simulink library "HardwareCommunication"  (R2016b)
settings: Solver=VariableStepAuto  StartTime=0.0  StopTime=10.0  RelTol=1e-3
undefined symbols (not defined in the file or in its folder): EthercatDeviceError
libraries: inSOMANET x28, SendToSOMANET x28, VariousLibrary x14, GESHandler x8, InputDeviceHandler x8, PDBHandler x8, SOMANETHandler x8, xpcethercatlib x7, ReceiveFromInputDevice x7, ReceiveFromGES x7, ReceiveFromPDB x7, SendToInputDevice x7
(part 1 of 2)
settings Model: Creator=march  LastModifiedBy=march

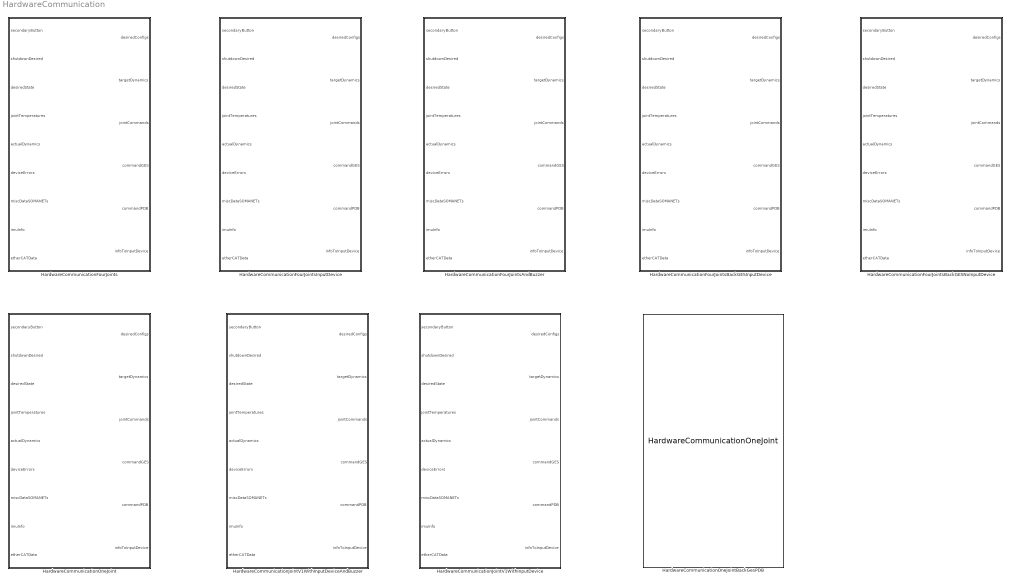
== system HardwareCommunication ==
  HardwareCommunicationFourJoints : Subsystem
  HardwareCommunicationFourJointsAndBuzzer : Subsystem
  HardwareCommunicationFourJointsBackGESInputDevice : Subsystem
  HardwareCommunicationFourJointsBackGESNoInputDevice : Subsystem
  HardwareCommunicationFourJointsInputDevice : Subsystem
  HardwareCommunicationJointV1WithInputDevice : Subsystem
  HardwareCommunicationJointV1WithInputDeviceAndBuzzer : Subsystem
  HardwareCommunicationOneJoint : Subsystem
  HardwareCommunicationOneJointBackGesPDB : HardwareCommunication/HardwareCommunicationOneJoint

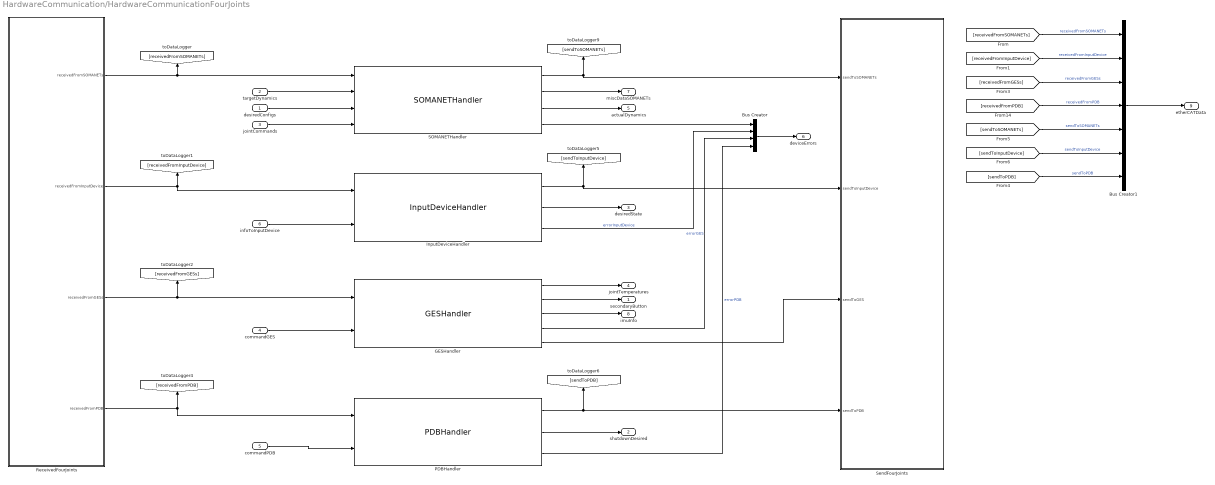
== system HardwareCommunication/HardwareCommunicationFourJoints ==
  desiredConfigs : Inport
  targetDynamics : Inport  Port=2
  jointCommands : Inport  Port=3
  commandGES : Inport  Port=4  OutDataTypeStr=Bus: commandGES
  commandPDB : Inport  Port=5
  infoToInputDevice : Inport  Port=6
  Bus Creator : BusCreator  Inputs=4  OutDataTypeStr=Bus: DeviceErrors  NonVirtualBus=on
  Bus Creator1 : BusCreator  Inputs=7  OutDataTypeStr=Bus: EtherCATData  NonVirtualBus=on
  GESHandler : GESHandler/GESHandler
  InputDeviceHandler : InputDeviceHandler/InputDeviceHandler
  PDBHandler : PDBHandler/PDBHandler
  ReceivedFourJoints : Subsystem
  SOMANETHandler : SOMANETHandler/SOMANETHandler
  SendFourJoints : Subsystem
  secondaryButton : Outport
  shutdownDesired : Outport  Port=2
  desiredState : Outport  Port=3
  jointTemperatures : Outport  Port=4
  actualDynamics : Outport  Port=5
  deviceErrors : Outport  Port=6
  miscDataSOMANETs : Outport  Port=7
  imuInfo : Outport  Port=8
  etherCATData : Outport  Port=9
  wires:
  GESHandler/5 -> SendFourJoints/3(sendToGES)
  infoToInputDevice/1 -> InputDeviceHandler/2
  ReceivedFourJoints/3(receivedFromGESs) -> GESHandler/1, [receivedFromGESs]
  ReceivedFourJoints/2(receivedFromInputDevice) -> InputDeviceHandler/1, [receivedFromInputDevice]
  ReceivedFourJoints/4(receivedFromPDB) -> PDBHandler/1, [receivedFromPDB]
  InputDeviceHandler/1 -> SendFourJoints/2(sendToInputDevice), [sendToInputDevice]
  InputDeviceHandler/3 -> Bus Creator/2  "errorInputDevice"
  Bus Creator/1 -> deviceErrors/1
  PDBHandler/1 -> SendFourJoints/4(sendToPDB), [sendToPDB]
  [receivedFromInputDevice] -> Bus Creator1/2  "receivedFromInputDevice"
  [receivedFromSOMANETs] -> Bus Creator1/1  "receivedFromSOMANETs"
  SOMANETHandler/2 -> miscDataSOMANETs/1
  [sendToPDB] -> Bus Creator1/7  "sendToPDB"
  ReceivedFourJoints/1(receivedFromSOMANETs) -> [receivedFromSOMANETs], SOMANETHandler/1
  GESHandler/2 -> secondaryButton/1
  SOMANETHandler/1 -> SendFourJoints/1(sendToSOMANETs), [sendToSOMANETs]
  InputDeviceHandler/2 -> desiredState/1
  jointCommands/1 -> SOMANETHandler/4
  SOMANETHandler/3 -> actualDynamics/1
  [sendToSOMANETs] -> Bus Creator1/5  "sendToSOMANETs"
  [sendToInputDevice] -> Bus Creator1/6  "sendToInputDevice"
  [receivedFromGESs] -> Bus Creator1/3  "receivedFromGESs"
  SOMANETHandler/4 -> Bus Creator/1
  desiredConfigs/1 -> SOMANETHandler/3
  [receivedFromPDB] -> Bus Creator1/4  "receivedFromPDB"
  Bus Creator1/1 -> etherCATData/1
  GESHandler/1 -> jointTemperatures/1
  PDBHandler/3 -> Bus Creator/4  "errorPDB"
  commandGES/1 -> GESHandler/2
  GESHandler/4 -> Bus Creator/3  "errorGES"
  commandPDB/1 -> PDBHandler/2
  PDBHandler/2 -> shutdownDesired/1
  targetDynamics/1 -> SOMANETHandler/2
  GESHandler/3 -> imuInfo/1

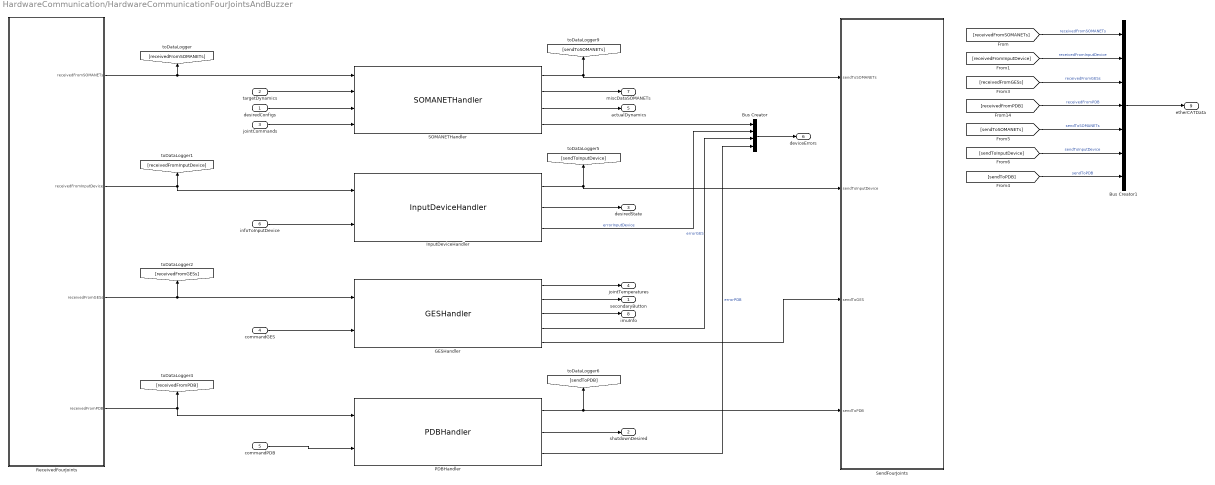
== system HardwareCommunication/HardwareCommunicationFourJointsAndBuzzer ==
  desiredConfigs : Inport
  targetDynamics : Inport  Port=2
  jointCommands : Inport  Port=3
  commandGES : Inport  Port=4
  commandPDB : Inport  Port=5
  infoToInputDevice : Inport  Port=6
  Bus Creator : BusCreator  Inputs=4  OutDataTypeStr=Bus: DeviceErrors  NonVirtualBus=on
  Bus Creator1 : BusCreator  Inputs=7  OutDataTypeStr=Bus: EtherCATData  NonVirtualBus=on
  GESHandler : GESHandler/GESHandler
  InputDeviceHandler : InputDeviceHandler/InputDeviceHandler
  PDBHandler : PDBHandler/PDBHandler
  ReceivedFourJoints : Subsystem
  SOMANETHandler : SOMANETHandler/SOMANETHandler
  SendFourJoints : Subsystem
  secondaryButton : Outport
  shutdownDesired : Outport  Port=2
  desiredState : Outport  Port=3
  jointTemperatures : Outport  Port=4
  actualDynamics : Outport  Port=5
  deviceErrors : Outport  Port=6
  miscDataSOMANETs : Outport  Port=7
  imuInfo : Outport  Port=8
  etherCATData : Outport  Port=9
  wires:
  GESHandler/5 -> SendFourJoints/3(sendToGES)
  infoToInputDevice/1 -> InputDeviceHandler/2
  ReceivedFourJoints/3(receivedFromGESs) -> GESHandler/1, [receivedFromGESs]
  ReceivedFourJoints/2(receivedFromInputDevice) -> InputDeviceHandler/1, [receivedFromInputDevice]
  ReceivedFourJoints/4(receivedFromPDB) -> PDBHandler/1, [receivedFromPDB]
  InputDeviceHandler/1 -> SendFourJoints/2(sendToInputDevice), [sendToInputDevice]
  InputDeviceHandler/3 -> Bus Creator/2  "errorInputDevice"
  Bus Creator/1 -> deviceErrors/1
  PDBHandler/1 -> SendFourJoints/4(sendToPDB), [sendToPDB]
  [receivedFromInputDevice] -> Bus Creator1/2  "receivedFromInputDevice"
  [receivedFromSOMANETs] -> Bus Creator1/1  "receivedFromSOMANETs"
  SOMANETHandler/2 -> miscDataSOMANETs/1
  [sendToPDB] -> Bus Creator1/7  "sendToPDB"
  ReceivedFourJoints/1(receivedFromSOMANETs) -> [receivedFromSOMANETs], SOMANETHandler/1
  GESHandler/2 -> secondaryButton/1
  SOMANETHandler/1 -> SendFourJoints/1(sendToSOMANETs), [sendToSOMANETs]
  InputDeviceHandler/2 -> desiredState/1
  jointCommands/1 -> SOMANETHandler/4
  SOMANETHandler/3 -> actualDynamics/1
  [sendToSOMANETs] -> Bus Creator1/5  "sendToSOMANETs"
  [sendToInputDevice] -> Bus Creator1/6  "sendToInputDevice"
  [receivedFromGESs] -> Bus Creator1/3  "receivedFromGESs"
  SOMANETHandler/4 -> Bus Creator/1
  desiredConfigs/1 -> SOMANETHandler/3
  [receivedFromPDB] -> Bus Creator1/4  "receivedFromPDB"
  Bus Creator1/1 -> etherCATData/1
  GESHandler/1 -> jointTemperatures/1
  PDBHandler/3 -> Bus Creator/4  "errorPDB"
  commandGES/1 -> GESHandler/2
  GESHandler/4 -> Bus Creator/3  "errorGES"
  commandPDB/1 -> PDBHandler/2
  PDBHandler/2 -> shutdownDesired/1
  targetDynamics/1 -> SOMANETHandler/2
  GESHandler/3 -> imuInfo/1

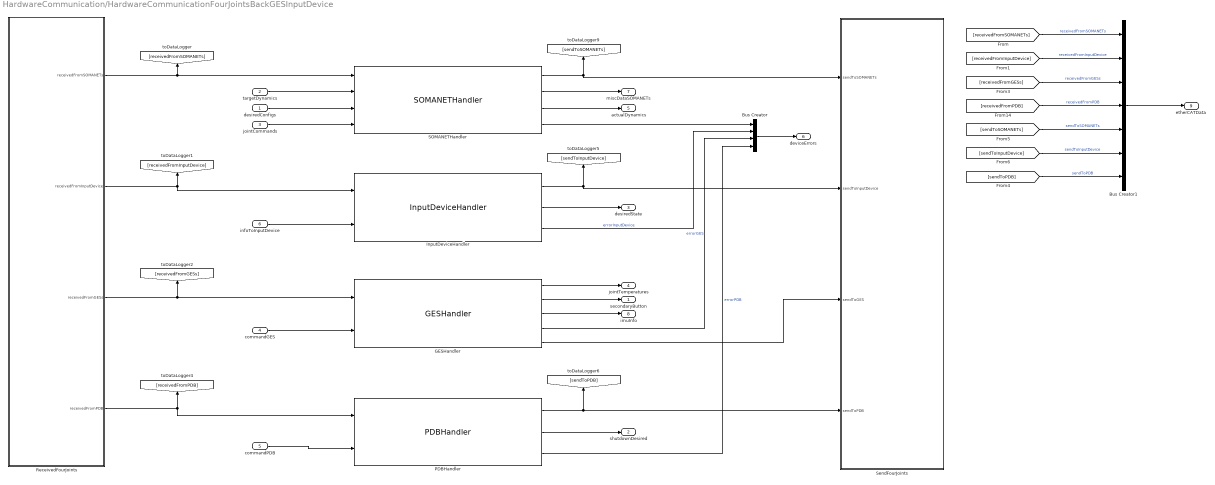
== system HardwareCommunication/HardwareCommunicationFourJointsBackGESInputDevice ==
  desiredConfigs : Inport
  targetDynamics : Inport  Port=2
  jointCommands : Inport  Port=3
  commandGES : Inport  Port=4
  commandPDB : Inport  Port=5
  infoToInputDevice : Inport  Port=6
  Bus Creator : BusCreator  Inputs=4  OutDataTypeStr=Bus: DeviceErrors  NonVirtualBus=on
  Bus Creator1 : BusCreator  Inputs=7  OutDataTypeStr=Bus: EtherCATData  NonVirtualBus=on
  GESHandler : GESHandler/GESHandler
  InputDeviceHandler : InputDeviceHandler/InputDeviceHandler
  PDBHandler : PDBHandler/PDBHandler
  ReceivedFourJoints : Subsystem
  SOMANETHandler : SOMANETHandler/SOMANETHandler
  SendFourJoints : Subsystem
  secondaryButton : Outport
  shutdownDesired : Outport  Port=2
  desiredState : Outport  Port=3
  jointTemperatures : Outport  Port=4
  actualDynamics : Outport  Port=5
  deviceErrors : Outport  Port=6
  miscDataSOMANETs : Outport  Port=7
  imuInfo : Outport  Port=8
  etherCATData : Outport  Port=9
  wires:
  GESHandler/3 -> imuInfo/1
  targetDynamics/1 -> SOMANETHandler/2
  PDBHandler/2 -> shutdownDesired/1
  commandPDB/1 -> PDBHandler/2
  GESHandler/4 -> Bus Creator/3  "errorGES"
  commandGES/1 -> GESHandler/2
  PDBHandler/3 -> Bus Creator/4  "errorPDB"
  GESHandler/1 -> jointTemperatures/1
  Bus Creator1/1 -> etherCATData/1
  [receivedFromPDB] -> Bus Creator1/4  "receivedFromPDB"
  desiredConfigs/1 -> SOMANETHandler/3
  SOMANETHandler/4 -> Bus Creator/1
  [receivedFromGESs] -> Bus Creator1/3  "receivedFromGESs"
  [sendToInputDevice] -> Bus Creator1/6  "sendToInputDevice"
  [sendToSOMANETs] -> Bus Creator1/5  "sendToSOMANETs"
  SOMANETHandler/3 -> actualDynamics/1
  jointCommands/1 -> SOMANETHandler/4
  InputDeviceHandler/2 -> desiredState/1
  SOMANETHandler/1 -> [sendToSOMANETs], SendFourJoints/1(sendToSOMANETs)
  GESHandler/2 -> secondaryButton/1
  ReceivedFourJoints/1(receivedFromSOMANETs) -> SOMANETHandler/1, [receivedFromSOMANETs]
  [sendToPDB] -> Bus Creator1/7  "sendToPDB"
  SOMANETHandler/2 -> miscDataSOMANETs/1
  [receivedFromSOMANETs] -> Bus Creator1/1  "receivedFromSOMANETs"
  [receivedFromInputDevice] -> Bus Creator1/2  "receivedFromInputDevice"
  PDBHandler/1 -> [sendToPDB], SendFourJoints/4(sendToPDB)
  Bus Creator/1 -> deviceErrors/1
  InputDeviceHandler/3 -> Bus Creator/2  "errorInputDevice"
  InputDeviceHandler/1 -> [sendToInputDevice], SendFourJoints/2(sendToInputDevice)
  ReceivedFourJoints/4(receivedFromPDB) -> [receivedFromPDB], PDBHandler/1
  ReceivedFourJoints/2(receivedFromInputDevice) -> [receivedFromInputDevice], InputDeviceHandler/1
  ReceivedFourJoints/3(receivedFromGESs) -> [receivedFromGESs], GESHandler/1
  infoToInputDevice/1 -> InputDeviceHandler/2
  GESHandler/5 -> SendFourJoints/3(sendToGES)

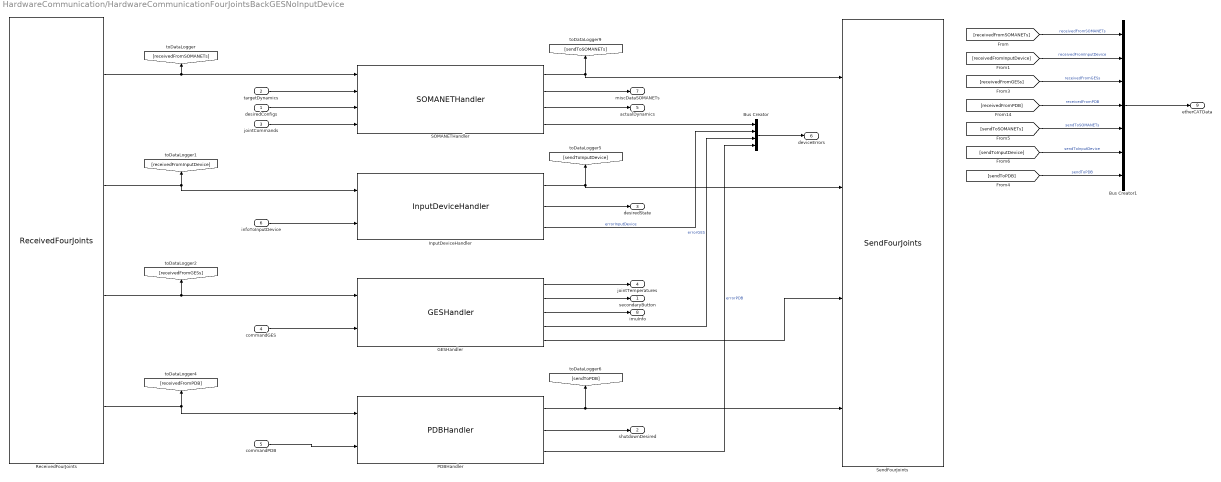
== system HardwareCommunication/HardwareCommunicationFourJointsBackGESNoInputDevice ==
  desiredConfigs : Inport
  targetDynamics : Inport  Port=2
  jointCommands : Inport  Port=3
  commandGES : Inport  Port=4
  commandPDB : Inport  Port=5
  infoToInputDevice : Inport  Port=6
  Bus Creator : BusCreator  Inputs=4  OutDataTypeStr=Bus: DeviceErrors  NonVirtualBus=on
  Bus Creator1 : BusCreator  Inputs=7  OutDataTypeStr=Bus: EtherCATData  NonVirtualBus=on
  GESHandler : GESHandler/GESHandler
  InputDeviceHandler : InputDeviceHandler/InputDeviceHandler
  PDBHandler : PDBHandler/PDBHandler
  ReceivedFourJoints : HardwareCommunication/HardwareCommunicationFourJointsBackGESInputDevice/ReceivedFourJoints
  SOMANETHandler : SOMANETHandler/SOMANETHandler
  SendFourJoints : HardwareCommunication/HardwareCommunicationFourJointsBackGESInputDevice/SendFourJoints
  secondaryButton : Outport
  shutdownDesired : Outport  Port=2
  desiredState : Outport  Port=3
  jointTemperatures : Outport  Port=4
  actualDynamics : Outport  Port=5
  deviceErrors : Outport  Port=6
  miscDataSOMANETs : Outport  Port=7
  imuInfo : Outport  Port=8
  etherCATData : Outport  Port=9
  wires:
  Bus Creator1/1 -> etherCATData/1
  desiredConfigs/1 -> SOMANETHandler/3
  SOMANETHandler/4 -> Bus Creator/1
  [receivedFromGESs] -> Bus Creator1/3  "receivedFromGESs"
  [receivedFromPDB] -> Bus Creator1/4  "receivedFromPDB"
  [sendToInputDevice] -> Bus Creator1/6  "sendToInputDevice"
  [sendToSOMANETs] -> Bus Creator1/5  "sendToSOMANETs"
  PDBHandler/3 -> Bus Creator/4  "errorPDB"
  SOMANETHandler/3 -> actualDynamics/1
  PDBHandler/2 -> shutdownDesired/1
  commandPDB/1 -> PDBHandler/2
  targetDynamics/1 -> SOMANETHandler/2
  GESHandler/4 -> Bus Creator/3  "errorGES"
  GESHandler/3 -> imuInfo/1
  commandGES/1 -> GESHandler/2
  GESHandler/1 -> jointTemperatures/1
  [receivedFromInputDevice] -> Bus Creator1/2  "receivedFromInputDevice"
  InputDeviceHandler/2 -> desiredState/1
  SOMANETHandler/1 -> [sendToSOMANETs], SendFourJoints/1
  InputDeviceHandler/1 -> [sendToInputDevice], SendFourJoints/2
  GESHandler/2 -> secondaryButton/1
  ReceivedFourJoints/2 -> [receivedFromInputDevice], InputDeviceHandler/1
  SOMANETHandler/2 -> miscDataSOMANETs/1
  PDBHandler/1 -> [sendToPDB], SendFourJoints/4
  [sendToPDB] -> Bus Creator1/7  "sendToPDB"
  Bus Creator/1 -> deviceErrors/1
  InputDeviceHandler/3 -> Bus Creator/2  "errorInputDevice"
  ReceivedFourJoints/4 -> [receivedFromPDB], PDBHandler/1
  GESHandler/5 -> SendFourJoints/3
  infoToInputDevice/1 -> InputDeviceHandler/2
  jointCommands/1 -> SOMANETHandler/4
  [receivedFromSOMANETs] -> Bus Creator1/1  "receivedFromSOMANETs"
  ReceivedFourJoints/1 -> SOMANETHandler/1, [receivedFromSOMANETs]
  ReceivedFourJoints/3 -> [receivedFromGESs], GESHandler/1

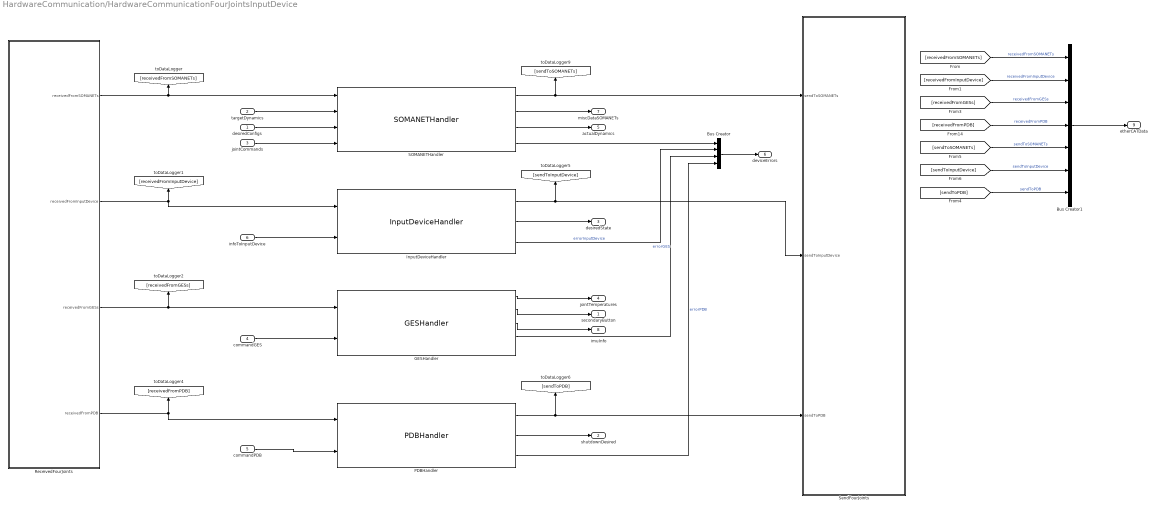
== system HardwareCommunication/HardwareCommunicationFourJointsInputDevice ==
  desiredConfigs : Inport
  targetDynamics : Inport  Port=2
  jointCommands : Inport  Port=3
  commandGES : Inport  Port=4
  commandPDB : Inport  Port=5
  infoToInputDevice : Inport  Port=6
  Bus Creator : BusCreator  Inputs=4  OutDataTypeStr=Bus: DeviceErrors  NonVirtualBus=on
  Bus Creator1 : BusCreator  Inputs=7  OutDataTypeStr=Bus: EtherCATData  NonVirtualBus=on
  GESHandler : GESHandler/GESHandler
  InputDeviceHandler : InputDeviceHandler/InputDeviceHandler
  PDBHandler : PDBHandler/PDBHandler
  ReceivedFourJoints : Subsystem
  SOMANETHandler : SOMANETHandler/SOMANETHandler
  SendFourJoints : Subsystem
  secondaryButton : Outport
  shutdownDesired : Outport  Port=2
  desiredState : Outport  Port=3
  jointTemperatures : Outport  Port=4
  actualDynamics : Outport  Port=5
  deviceErrors : Outport  Port=6
  miscDataSOMANETs : Outport  Port=7
  imuInfo : Outport  Port=8
  etherCATData : Outport  Port=9
  wires:
  GESHandler/3 -> imuInfo/1
  targetDynamics/1 -> SOMANETHandler/2
  PDBHandler/2 -> shutdownDesired/1
  commandPDB/1 -> PDBHandler/2
  GESHandler/4 -> Bus Creator/3  "errorGES"
  commandGES/1 -> GESHandler/2
  PDBHandler/3 -> Bus Creator/4  "errorPDB"
  GESHandler/1 -> jointTemperatures/1
  Bus Creator1/1 -> etherCATData/1
  [receivedFromPDB] -> Bus Creator1/4  "receivedFromPDB"
  desiredConfigs/1 -> SOMANETHandler/3
  SOMANETHandler/4 -> Bus Creator/1
  [receivedFromGESs] -> Bus Creator1/3  "receivedFromGESs"
  [sendToInputDevice] -> Bus Creator1/6  "sendToInputDevice"
  [sendToSOMANETs] -> Bus Creator1/5  "sendToSOMANETs"
  SOMANETHandler/3 -> actualDynamics/1
  jointCommands/1 -> SOMANETHandler/4
  InputDeviceHandler/2 -> desiredState/1
  SOMANETHandler/1 -> [sendToSOMANETs], SendFourJoints/1(sendToSOMANETs)
  GESHandler/2 -> secondaryButton/1
  ReceivedFourJoints/1(receivedFromSOMANETs) -> SOMANETHandler/1, [receivedFromSOMANETs]
  [sendToPDB] -> Bus Creator1/7  "sendToPDB"
  SOMANETHandler/2 -> miscDataSOMANETs/1
  [receivedFromSOMANETs] -> Bus Creator1/1  "receivedFromSOMANETs"
  [receivedFromInputDevice] -> Bus Creator1/2  "receivedFromInputDevice"
  PDBHandler/1 -> [sendToPDB], SendFourJoints/3(sendToPDB)
  Bus Creator/1 -> deviceErrors/1
  InputDeviceHandler/3 -> Bus Creator/2  "errorInputDevice"
  InputDeviceHandler/1 -> [sendToInputDevice], SendFourJoints/2(sendToInputDevice)
  ReceivedFourJoints/4(receivedFromPDB) -> [receivedFromPDB], PDBHandler/1
  ReceivedFourJoints/2(receivedFromInputDevice) -> [receivedFromInputDevice], InputDeviceHandler/1
  ReceivedFourJoints/3(receivedFromGESs) -> [receivedFromGESs], GESHandler/1
  infoToInputDevice/1 -> InputDeviceHandler/2

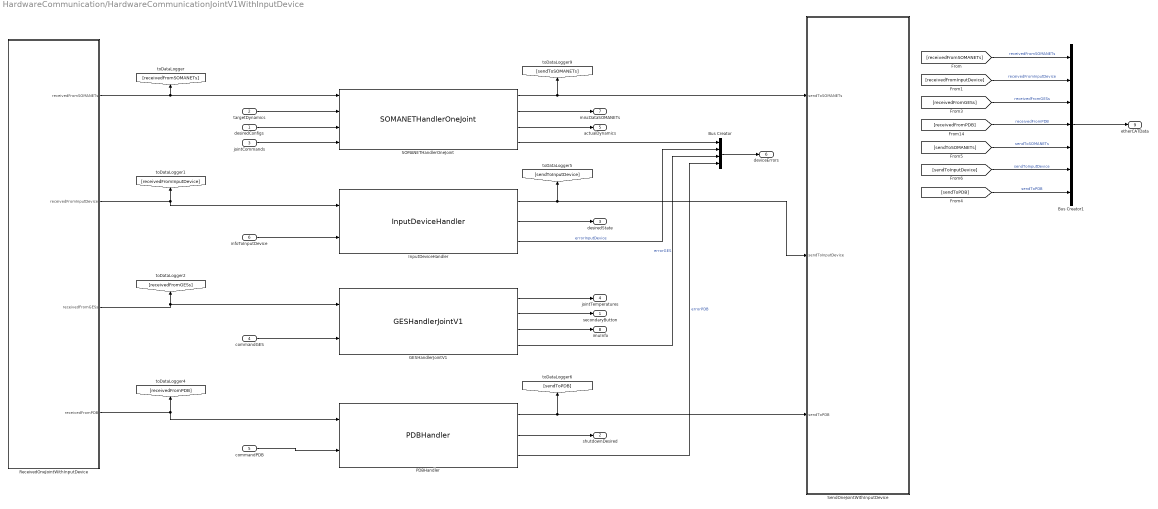
== system HardwareCommunication/HardwareCommunicationJointV1WithInputDevice ==
  desiredConfigs : Inport
  targetDynamics : Inport  Port=2
  jointCommands : Inport  Port=3
  commandGES : Inport  Port=4
  commandPDB : Inport  Port=5
  infoToInputDevice : Inport  Port=6
  Bus Creator : BusCreator  Inputs=4  OutDataTypeStr=Bus: DeviceErrors  NonVirtualBus=on
  Bus Creator1 : BusCreator  Inputs=7  OutDataTypeStr=Bus: EtherCATData  NonVirtualBus=on
  GESHandlerJointV1 : GESHandler/GESHandlerJointV1
  InputDeviceHandler : InputDeviceHandler/InputDeviceHandler
  PDBHandler : PDBHandler/PDBHandler
  ReceivedOneJointWithInputDevice : Subsystem
  SOMANETHandlerOneJoint : SOMANETHandler/SOMANETHandlerOneJoint
  SendOneJointWithInputDevice : Subsystem
  secondaryButton : Outport
  shutdownDesired : Outport  Port=2
  desiredState : Outport  Port=3
  jointTemperatures : Outport  Port=4
  actualDynamics : Outport  Port=5
  deviceErrors : Outport  Port=6
  miscDataSOMANETs : Outport  Port=7
  imuInfo : Outport  Port=8
  etherCATData : Outport  Port=9
  wires:
  infoToInputDevice/1 -> InputDeviceHandler/2
  ReceivedOneJointWithInputDevice/3(receivedFromGESs) -> [receivedFromGESs], GESHandlerJointV1/1
  ReceivedOneJointWithInputDevice/2(receivedFromInputDevice) -> InputDeviceHandler/1, [receivedFromInputDevice]
  ReceivedOneJointWithInputDevice/4(receivedFromPDB) -> PDBHandler/1, [receivedFromPDB]
  InputDeviceHandler/1 -> [sendToInputDevice], SendOneJointWithInputDevice/2(sendToInputDevice)
  InputDeviceHandler/3 -> Bus Creator/2  "errorInputDevice"
  Bus Creator/1 -> deviceErrors/1
  PDBHandler/1 -> [sendToPDB], SendOneJointWithInputDevice/3(sendToPDB)
  [receivedFromInputDevice] -> Bus Creator1/2  "receivedFromInputDevice"
  [receivedFromSOMANETs] -> Bus Creator1/1  "receivedFromSOMANETs"
  SOMANETHandlerOneJoint/2 -> miscDataSOMANETs/1
  [sendToPDB] -> Bus Creator1/7  "sendToPDB"
  ReceivedOneJointWithInputDevice/1(receivedFromSOMANETs) -> [receivedFromSOMANETs], SOMANETHandlerOneJoint/1
  GESHandlerJointV1/2 -> secondaryButton/1
  SOMANETHandlerOneJoint/1 -> [sendToSOMANETs], SendOneJointWithInputDevice/1(sendToSOMANETs)
  InputDeviceHandler/2 -> desiredState/1
  jointCommands/1 -> SOMANETHandlerOneJoint/4
  SOMANETHandlerOneJoint/3 -> actualDynamics/1
  [sendToSOMANETs] -> Bus Creator1/5  "sendToSOMANETs"
  [sendToInputDevice] -> Bus Creator1/6  "sendToInputDevice"
  [receivedFromGESs] -> Bus Creator1/3  "receivedFromGESs"
  SOMANETHandlerOneJoint/4 -> Bus Creator/1
  desiredConfigs/1 -> SOMANETHandlerOneJoint/3
  [receivedFromPDB] -> Bus Creator1/4  "receivedFromPDB"
  Bus Creator1/1 -> etherCATData/1
  GESHandlerJointV1/1 -> jointTemperatures/1
  PDBHandler/3 -> Bus Creator/4  "errorPDB"
  commandGES/1 -> GESHandlerJointV1/2
  GESHandlerJointV1/4 -> Bus Creator/3  "errorGES"
  commandPDB/1 -> PDBHandler/2
  PDBHandler/2 -> shutdownDesired/1
  targetDynamics/1 -> SOMANETHandlerOneJoint/2
  GESHandlerJointV1/3 -> imuInfo/1

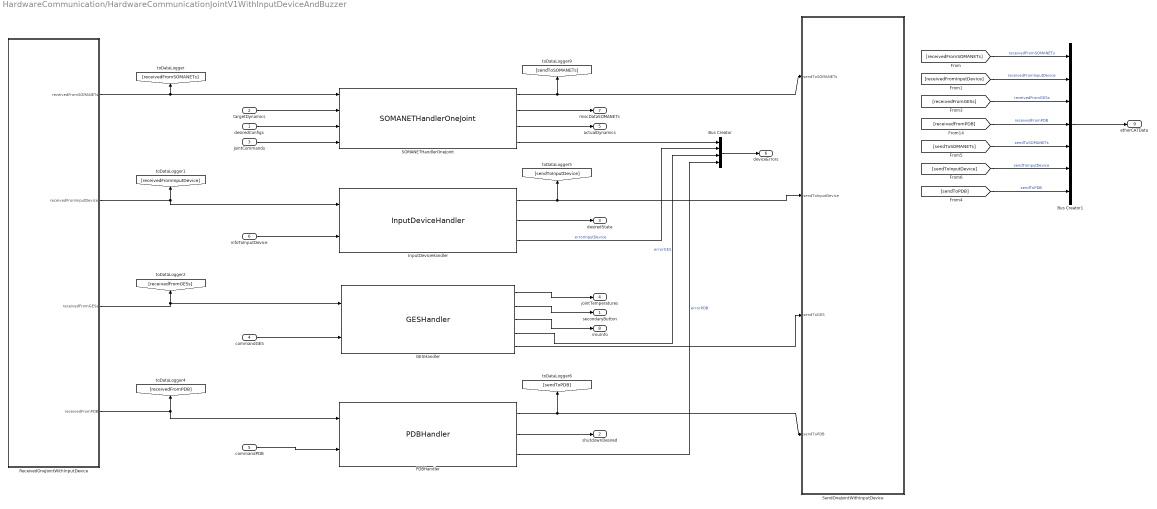
== system HardwareCommunication/HardwareCommunicationJointV1WithInputDeviceAndBuzzer ==
  desiredConfigs : Inport
  targetDynamics : Inport  Port=2
  jointCommands : Inport  Port=3
  commandGES : Inport  Port=4
  commandPDB : Inport  Port=5
  infoToInputDevice : Inport  Port=6
  Bus Creator : BusCreator  Inputs=4  OutDataTypeStr=Bus: DeviceErrors  NonVirtualBus=on
  Bus Creator1 : BusCreator  Inputs=7  OutDataTypeStr=Bus: EtherCATData  NonVirtualBus=on
  GESHandler : GESHandler/GESHandler
  InputDeviceHandler : InputDeviceHandler/InputDeviceHandler
  PDBHandler : PDBHandler/PDBHandler
  ReceivedOneJointWithInputDevice : Subsystem
  SOMANETHandlerOneJoint : SOMANETHandler/SOMANETHandlerOneJoint
  SendOneJointWithInputDevice : Subsystem
  secondaryButton : Outport
  shutdownDesired : Outport  Port=2
  desiredState : Outport  Port=3
  jointTemperatures : Outport  Port=4
  actualDynamics : Outport  Port=5
  deviceErrors : Outport  Port=6
  miscDataSOMANETs : Outport  Port=7
  imuInfo : Outport  Port=8
  etherCATData : Outport  Port=9
  wires:
  infoToInputDevice/1 -> InputDeviceHandler/2
  ReceivedOneJointWithInputDevice/3(receivedFromGESs) -> GESHandler/1, [receivedFromGESs]
  ReceivedOneJointWithInputDevice/2(receivedFromInputDevice) -> InputDeviceHandler/1, [receivedFromInputDevice]
  ReceivedOneJointWithInputDevice/4(receivedFromPDB) -> PDBHandler/1, [receivedFromPDB]
  InputDeviceHandler/1 -> [sendToInputDevice], SendOneJointWithInputDevice/2(sendToInputDevice)
  InputDeviceHandler/3 -> Bus Creator/2  "errorInputDevice"
  Bus Creator/1 -> deviceErrors/1
  PDBHandler/1 -> [sendToPDB], SendOneJointWithInputDevice/4(sendToPDB)
  [receivedFromInputDevice] -> Bus Creator1/2  "receivedFromInputDevice"
  [receivedFromSOMANETs] -> Bus Creator1/1  "receivedFromSOMANETs"
  SOMANETHandlerOneJoint/2 -> miscDataSOMANETs/1
  [sendToPDB] -> Bus Creator1/7  "sendToPDB"
  ReceivedOneJointWithInputDevice/1(receivedFromSOMANETs) -> [receivedFromSOMANETs], SOMANETHandlerOneJoint/1
  GESHandler/2 -> secondaryButton/1
  SOMANETHandlerOneJoint/1 -> [sendToSOMANETs], SendOneJointWithInputDevice/1(sendToSOMANETs)
  InputDeviceHandler/2 -> desiredState/1
  jointCommands/1 -> SOMANETHandlerOneJoint/4
  SOMANETHandlerOneJoint/3 -> actualDynamics/1
  [sendToSOMANETs] -> Bus Creator1/5  "sendToSOMANETs"
  [sendToInputDevice] -> Bus Creator1/6  "sendToInputDevice"
  [receivedFromGESs] -> Bus Creator1/3  "receivedFromGESs"
  SOMANETHandlerOneJoint/4 -> Bus Creator/1
  desiredConfigs/1 -> SOMANETHandlerOneJoint/3
  [receivedFromPDB] -> Bus Creator1/4  "receivedFromPDB"
  Bus Creator1/1 -> etherCATData/1
  GESHandler/1 -> jointTemperatures/1
  PDBHandler/3 -> Bus Creator/4  "errorPDB"
  commandGES/1 -> GESHandler/2
  GESHandler/4 -> Bus Creator/3  "errorGES"
  commandPDB/1 -> PDBHandler/2
  PDBHandler/2 -> shutdownDesired/1
  targetDynamics/1 -> SOMANETHandlerOneJoint/2
  GESHandler/3 -> imuInfo/1
  GESHandler/5 -> SendOneJointWithInputDevice/3(sendToGES)

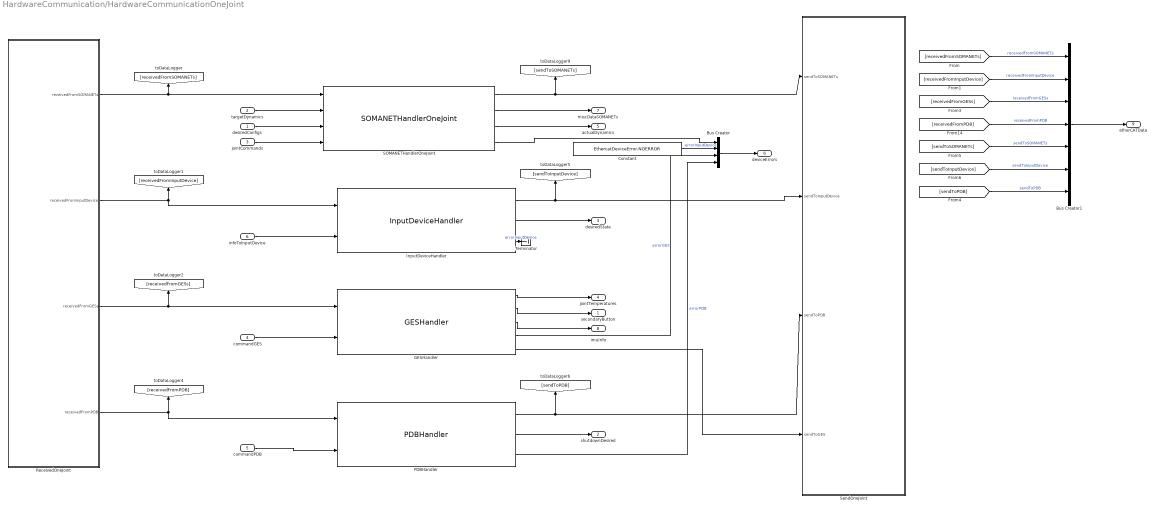
== system HardwareCommunication/HardwareCommunicationOneJoint ==
  desiredConfigs : Inport
  targetDynamics : Inport  Port=2
  jointCommands : Inport  Port=3
  commandGES : Inport  Port=4
  commandPDB : Inport  Port=5
  infoToInputDevice : Inport  Port=6
  Bus Creator : BusCreator  Inputs=4  OutDataTypeStr=Bus: DeviceErrors  NonVirtualBus=on
  Bus Creator1 : BusCreator  Inputs=7  OutDataTypeStr=Bus: EtherCATData  NonVirtualBus=on
  Constant : Constant  Value=EthercatDeviceError.NOERROR
  GESHandler : GESHandler/GESHandler
  InputDeviceHandler : InputDeviceHandler/InputDeviceHandler
  PDBHandler : PDBHandler/PDBHandler
  ReceivedOneJoint : Subsystem
  SOMANETHandlerOneJoint : SOMANETHandler/SOMANETHandlerOneJoint
  SendOneJoint : Subsystem
  Terminator : Terminator
  secondaryButton : Outport
  shutdownDesired : Outport  Port=2
  desiredState : Outport  Port=3
  jointTemperatures : Outport  Port=4
  actualDynamics : Outport  Port=5
  deviceErrors : Outport  Port=6
  miscDataSOMANETs : Outport  Port=7
  imuInfo : Outport  Port=8
  etherCATData : Outport  Port=9
  wires:
  InputDeviceHandler/3 -> Terminator/1  "errorInputDevice"
  Constant/1 -> Bus Creator/2  "errorInputDevice"
  GESHandler/5 -> SendOneJoint/4(sendToGES)
  infoToInputDevice/1 -> InputDeviceHandler/2
  ReceivedOneJoint/3(receivedFromGESs) -> GESHandler/1, [receivedFromGESs]
  ReceivedOneJoint/2(receivedFromInputDevice) -> InputDeviceHandler/1, [receivedFromInputDevice]
  ReceivedOneJoint/4(receivedFromPDB) -> PDBHandler/1, [receivedFromPDB]
  InputDeviceHandler/1 -> SendOneJoint/2(sendToInputDevice), [sendToInputDevice]
  Bus Creator/1 -> deviceErrors/1
  PDBHandler/1 -> SendOneJoint/3(sendToPDB), [sendToPDB]
  [receivedFromInputDevice] -> Bus Creator1/2  "receivedFromInputDevice"
  [receivedFromSOMANETs] -> Bus Creator1/1  "receivedFromSOMANETs"
  SOMANETHandlerOneJoint/2 -> miscDataSOMANETs/1
  [sendToPDB] -> Bus Creator1/7  "sendToPDB"
  ReceivedOneJoint/1(receivedFromSOMANETs) -> [receivedFromSOMANETs], SOMANETHandlerOneJoint/1
  GESHandler/2 -> secondaryButton/1
  SOMANETHandlerOneJoint/1 -> SendOneJoint/1(sendToSOMANETs), [sendToSOMANETs]
  InputDeviceHandler/2 -> desiredState/1
  jointCommands/1 -> SOMANETHandlerOneJoint/4
  SOMANETHandlerOneJoint/3 -> actualDynamics/1
  [sendToSOMANETs] -> Bus Creator1/5  "sendToSOMANETs"
  [sendToInputDevice] -> Bus Creator1/6  "sendToInputDevice"
  [receivedFromGESs] -> Bus Creator1/3  "receivedFromGESs"
  SOMANETHandlerOneJoint/4 -> Bus Creator/1
  desiredConfigs/1 -> SOMANETHandlerOneJoint/3
  [receivedFromPDB] -> Bus Creator1/4  "receivedFromPDB"
  Bus Creator1/1 -> etherCATData/1
  GESHandler/1 -> jointTemperatures/1
  PDBHandler/3 -> Bus Creator/4  "errorPDB"
  commandGES/1 -> GESHandler/2
  GESHandler/4 -> Bus Creator/3  "errorGES"
  commandPDB/1 -> PDBHandler/2
  PDBHandler/2 -> shutdownDesired/1
  targetDynamics/1 -> SOMANETHandlerOneJoint/2
  GESHandler/3 -> imuInfo/1

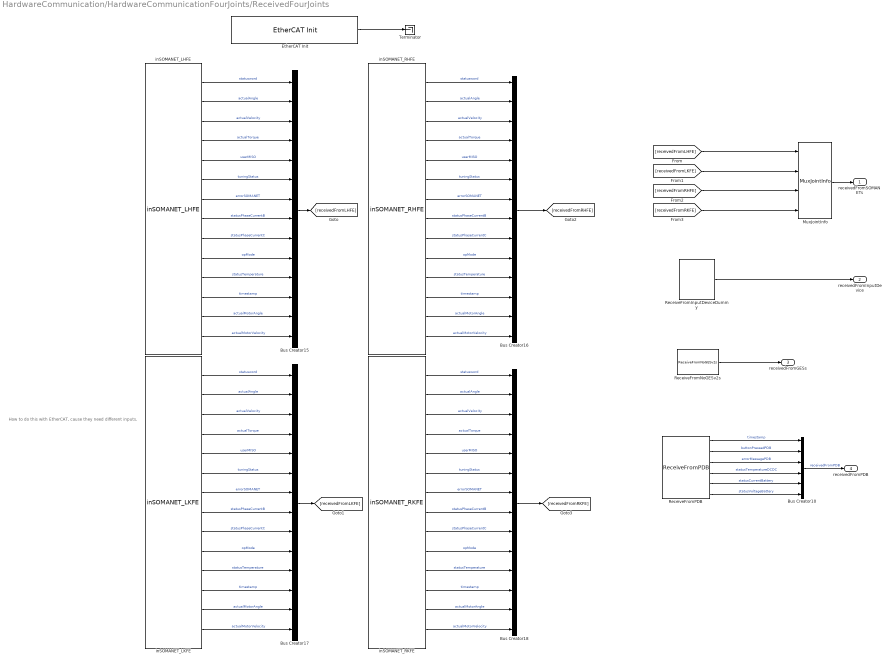
== system HardwareCommunication/HardwareCommunicationFourJoints/ReceivedFourJoints ==
  note: How to do this with EtherCAT, cause they need different inputs.
  Bus Creator10 : BusCreator  Inputs=6  OutDataTypeStr=Bus: EtherCATReceivedFromPDB  NonVirtualBus=on
  Bus Creator{15..18} (4 alike) : BusCreator  Inputs=14  OutDataTypeStr=Bus: EtherCATReceivedFromSOMANET  NonVirtualBus=on
  "EtherCAT Init " : xpcethercatlib/EtherCAT Init   Priority=0  config_file=..\EcatXML\FourJointsOnly_eni.xml  device_id=0  pci_bus=2  pci_slot=0  dctuning=0  enaDebug=on  enaDC=on  errLink=on  masterDbg=on  stateChgDbg=on  baseClock=off  masterCfg=off  logFile='c:\dbglog.txt'  sample_time=0.002000  DCMode=0
  MuxJointInfo : VariousLibrary/MuxJointInfo
  ReceiveFromInputDeviceDummy : ReceiveFromInputDevice/ReceiveFromInputDeviceDummy
  ReceiveFromNoGESv2s : ReceiveFromGES/ReceiveFromNoGESv2s
  ReceiveFromPDB : ReceiveFromPDB/ReceiveFromPDB
  Terminator : Terminator
  inSOMANET_LHFE : inSOMANET/inSOMANET_LHFE
  inSOMANET_LKFE : inSOMANET/inSOMANET_LKFE
  inSOMANET_RHFE : inSOMANET/inSOMANET_RHFE
  inSOMANET_RKFE : inSOMANET/inSOMANET_RKFE
  receivedFromSOMANETs : Outport  OutDataTypeStr=Bus: EtherCATReceivedFromSOMANET  PortDimensions=[ 1 4 ]  BusOutputAsStruct=on
  receivedFromInputDevice : Outport  Port=2  OutDataTypeStr=Bus: EtherCATReceivedFromInputDevice  BusOutputAsStruct=on
  receivedFromGESs : Outport  Port=3  OutDataTypeStr=Bus: EtherCATReceivedFromGES  PortDimensions=[1 4]  BusOutputAsStruct=on
  receivedFromPDB : Outport  Port=4  OutDataTypeStr=Bus: EtherCATReceivedFromPDB  BusOutputAsStruct=on
  wires:
  ReceiveFromPDB/1 -> Bus Creator10/1  "timestamp"
  [receivedFromLKFE] -> MuxJointInfo/2
  [receivedFromRKFE] -> MuxJointInfo/4
  [receivedFromRHFE] -> MuxJointInfo/3
  [receivedFromLHFE] -> MuxJointInfo/1
  Bus Creator18/1 -> [receivedFromRKFE]
  inSOMANET_RKFE/11 -> Bus Creator18/11  "statusTemperature"
  inSOMANET_LKFE/11 -> Bus Creator17/11  "statusTemperature"
  inSOMANET_RKFE/12 -> Bus Creator18/12  "timestamp"
  inSOMANET_RKFE/6 -> Bus Creator18/6  "tuningStatus"
  inSOMANET_RKFE/1 -> Bus Creator18/1  "statusword"
  inSOMANET_LKFE/5 -> Bus Creator17/5  "userMISO"
  inSOMANET_RKFE/7 -> Bus Creator18/7  "errorSOMANET"
  inSOMANET_RKFE/8 -> Bus Creator18/8  "statusPhaseCurrentB"
  inSOMANET_RKFE/3 -> Bus Creator18/3  "actualVelocity"
  inSOMANET_RKFE/5 -> Bus Creator18/5  "userMISO"
  inSOMANET_LKFE/8 -> Bus Creator17/8  "statusPhaseCurrentB"
  inSOMANET_LKFE/12 -> Bus Creator17/12  "timestamp"
  Bus Creator17/1 -> [receivedFromLKFE]
  inSOMANET_RKFE/10 -> Bus Creator18/10  "opMode"
  inSOMANET_LKFE/6 -> Bus Creator17/6  "tuningStatus"
  inSOMANET_LKFE/10 -> Bus Creator17/10  "opMode"
  inSOMANET_RKFE/2 -> Bus Creator18/2  "actualAngle"
  inSOMANET_RKFE/9 -> Bus Creator18/9  "statusPhaseCurrentC"
  inSOMANET_RKFE/4 -> Bus Creator18/4  "actualTorque"
  inSOMANET_LKFE/9 -> Bus Creator17/9  "statusPhaseCurrentC"
  inSOMANET_LHFE/9 -> Bus Creator15/9  "statusPhaseCurrentC"
  inSOMANET_LKFE/7 -> Bus Creator17/7  "errorSOMANET"
  inSOMANET_LKFE/4 -> Bus Creator17/4  "actualTorque"
  MuxJointInfo/1 -> receivedFromSOMANETs/1
  inSOMANET_LKFE/3 -> Bus Creator17/3  "actualVelocity"
  inSOMANET_RHFE/8 -> Bus Creator16/8  "statusPhaseCurrentB"
  inSOMANET_RHFE/5 -> Bus Creator16/5  "userMISO"
  inSOMANET_LHFE/8 -> Bus Creator15/8  "statusPhaseCurrentB"
  inSOMANET_LHFE/4 -> Bus Creator15/4  "actualTorque"
  inSOMANET_LHFE/12 -> Bus Creator15/12  "timestamp"
  inSOMANET_LKFE/2 -> Bus Creator17/2  "actualAngle"
  inSOMANET_RHFE/12 -> Bus Creator16/12  "timestamp"
  inSOMANET_LHFE/3 -> Bus Creator15/3  "actualVelocity"
  inSOMANET_LKFE/1 -> Bus Creator17/1  "statusword"
  Bus Creator16/1 -> [receivedFromRHFE]
  Bus Creator15/1 -> [receivedFromLHFE]
  inSOMANET_RHFE/11 -> Bus Creator16/11  "statusTemperature"
  inSOMANET_LHFE/7 -> Bus Creator15/7  "errorSOMANET"
  inSOMANET_RHFE/10 -> Bus Creator16/10  "opMode"
  inSOMANET_RHFE/9 -> Bus Creator16/9  "statusPhaseCurrentC"
  inSOMANET_RHFE/7 -> Bus Creator16/7  "errorSOMANET"
  inSOMANET_RHFE/1 -> Bus Creator16/1  "statusword"
  inSOMANET_LHFE/2 -> Bus Creator15/2  "actualAngle"
  inSOMANET_RHFE/6 -> Bus Creator16/6  "tuningStatus"
  inSOMANET_RHFE/4 -> Bus Creator16/4  "actualTorque"
  inSOMANET_RHFE/3 -> Bus Creator16/3  "actualVelocity"
  inSOMANET_RHFE/2 -> Bus Creator16/2  "actualAngle"
  inSOMANET_LHFE/11 -> Bus Creator15/11  "statusTemperature"
  inSOMANET_LHFE/1 -> Bus Creator15/1  "statusword"
  inSOMANET_LHFE/10 -> Bus Creator15/10  "opMode"
  inSOMANET_LHFE/6 -> Bus Creator15/6  "tuningStatus"
  Bus Creator10/1 -> receivedFromPDB/1  "receivedFromPDB"
  inSOMANET_LHFE/5 -> Bus Creator15/5  "userMISO"
  "EtherCAT Init "/1 -> Terminator/1
  inSOMANET_LHFE/13 -> Bus Creator15/13  "actualMotorAngle"
  inSOMANET_LHFE/14 -> Bus Creator15/14  "actualMotorVelocity"
  inSOMANET_LKFE/13 -> Bus Creator17/13  "actualMotorAngle"
  inSOMANET_LKFE/14 -> Bus Creator17/14  "actualMotorVelocity"
  inSOMANET_RKFE/13 -> Bus Creator18/13  "actualMotorAngle"
  inSOMANET_RKFE/14 -> Bus Creator18/14  "actualMotorVelocity"
  inSOMANET_RHFE/13 -> Bus Creator16/13  "actualMotorAngle"
  inSOMANET_RHFE/14 -> Bus Creator16/14  "actualMotorVelocity"
  ReceiveFromNoGESv2s/1 -> receivedFromGESs/1
  ReceiveFromPDB/3 -> Bus Creator10/3  "errorMessagePDB"
  ReceiveFromPDB/4 -> Bus Creator10/4  "statusTemperatureDCDC"
  ReceiveFromPDB/5 -> Bus Creator10/5  "statusCurrentBattery"
  ReceiveFromPDB/6 -> Bus Creator10/6  "statusVoltageBattery"
  ReceiveFromPDB/2 -> Bus Creator10/2  "buttonPressedPDB"
  ReceiveFromInputDeviceDummy/1 -> receivedFromInputDevice/1

== system HardwareCommunication/HardwareCommunicationFourJoints/SendFourJoints ==
  sendToSOMANETs : Inport  OutDataTypeStr=Bus: EtherCATSendToSOMANET  PortDimensions=[1 4]  BusOutputAsStruct=on
  sendToInputDevice : Inport  Port=2  OutDataTypeStr=Bus: EtherCATSendToInputDevice  BusOutputAsStruct=on
  sendToGES : Inport  Port=3  OutDataTypeStr=Bus: commandGES  BusOutputAsStruct=on
  sendToPDB : Inport  Port=4  OutDataTypeStr=Bus: EtherCATSendToPDB  BusOutputAsStruct=on
  Bus Selector10 : BusSelector  OutputSignals=masterState,errorMessage
  DemuxJointInfo : VariousLibrary/DemuxJointInfo
  "SendToInputDeviceDummy " : SendToInputDevice/SendToInputDeviceDummy 
  SendToPDB : SendToPDB/SendToPDB
  SendToSomanetLHFE : SendToSOMANET/SendToSomanetLHFE
  SendToSomanetLKFE : SendToSOMANET/SendToSomanetLKFE
  SendToSomanetRHFE : SendToSOMANET/SendToSomanetRHFE
  SendToSomanetRKFE : SendToSOMANET/SendToSomanetRKFE
  "sendToGESDummy " : SendToGES/sendToGESDummy 
  wires:
  sendToGES/1 -> "sendToGESDummy "/1
  sendToInputDevice/1 -> Bus Selector10/1
  DemuxJointInfo/4 -> SendToSomanetRKFE/1
  Bus Selector10/1 -> "SendToInputDeviceDummy "/1  "<masterState>"
  Bus Selector10/2 -> "SendToInputDeviceDummy "/2  "<errorMessage>"
  DemuxJointInfo/1 -> SendToSomanetLHFE/1
  DemuxJointInfo/2 -> SendToSomanetLKFE/1
  DemuxJointInfo/3 -> SendToSomanetRHFE/1
  sendToSOMANETs/1 -> DemuxJointInfo/1
  sendToPDB/1 -> SendToPDB/1

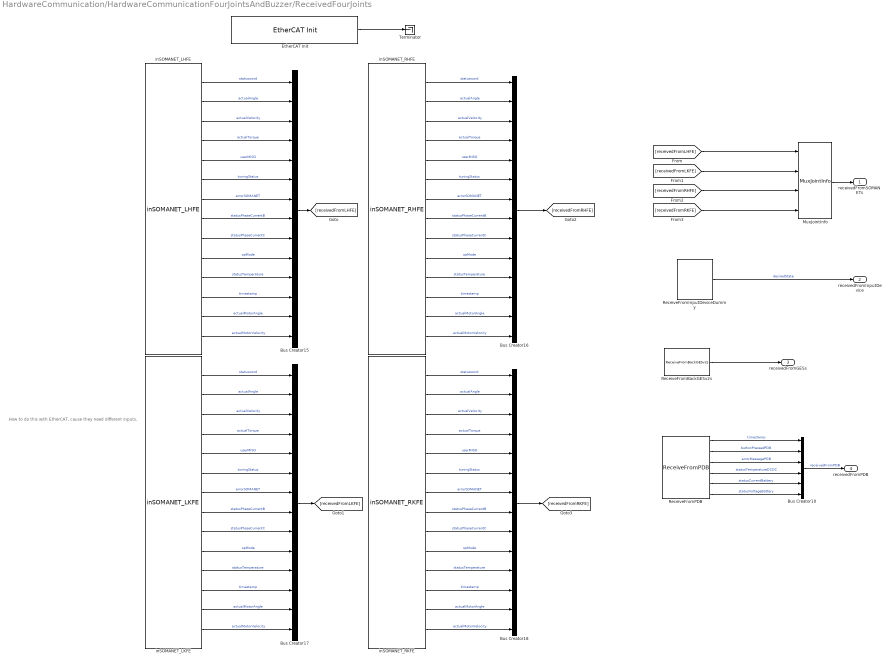
== system HardwareCommunication/HardwareCommunicationFourJointsAndBuzzer/ReceivedFourJoints ==
  note: How to do this with EtherCAT, cause they need different inputs.
  Bus Creator10 : BusCreator  Inputs=6  OutDataTypeStr=Bus: EtherCATReceivedFromPDB  NonVirtualBus=on
  Bus Creator{15..18} (4 alike) : BusCreator  Inputs=14  OutDataTypeStr=Bus: EtherCATReceivedFromSOMANET  NonVirtualBus=on
  "EtherCAT Init " : xpcethercatlib/EtherCAT Init   Priority=0  config_file=..\EcatXML\FourJointsWithGESBack.xml  device_id=0  pci_bus=2  pci_slot=0  dctuning=0  enaDebug=on  enaDC=on  errLink=on  masterDbg=on  stateChgDbg=on  baseClock=off  masterCfg=off  logFile='c:\dbglog.txt'  sample_time=0.002000  DCMode=0
  MuxJointInfo : VariousLibrary/MuxJointInfo
  ReceiveFromBackGESv2s : ReceiveFromGES/ReceiveFromBackGESv2s
  ReceiveFromInputDeviceDummy : ReceiveFromInputDevice/ReceiveFromInputDeviceDummy
  ReceiveFromPDB : ReceiveFromPDB/ReceiveFromPDB
  Terminator : Terminator
  inSOMANET_LHFE : inSOMANET/inSOMANET_LHFE
  inSOMANET_LKFE : inSOMANET/inSOMANET_LKFE
  inSOMANET_RHFE : inSOMANET/inSOMANET_RHFE
  inSOMANET_RKFE : inSOMANET/inSOMANET_RKFE
  receivedFromSOMANETs : Outport  OutDataTypeStr=Bus: EtherCATReceivedFromSOMANET  PortDimensions=[ 1 4 ]  BusOutputAsStruct=on
  receivedFromInputDevice : Outport  Port=2  OutDataTypeStr=Bus: EtherCATReceivedFromInputDevice  BusOutputAsStruct=on
  receivedFromGESs : Outport  Port=3  OutDataTypeStr=Bus: EtherCATReceivedFromGES  PortDimensions=[1 4]  BusOutputAsStruct=on
  receivedFromPDB : Outport  Port=4  OutDataTypeStr=Bus: EtherCATReceivedFromPDB  BusOutputAsStruct=on
  wires:
  ReceiveFromPDB/1 -> Bus Creator10/1  "timestamp"
  [receivedFromLKFE] -> MuxJointInfo/2
  [receivedFromRKFE] -> MuxJointInfo/4
  [receivedFromRHFE] -> MuxJointInfo/3
  [receivedFromLHFE] -> MuxJointInfo/1
  Bus Creator18/1 -> [receivedFromRKFE]
  inSOMANET_RKFE/11 -> Bus Creator18/11  "statusTemperature"
  inSOMANET_LKFE/11 -> Bus Creator17/11  "statusTemperature"
  inSOMANET_RKFE/12 -> Bus Creator18/12  "timestamp"
  inSOMANET_RKFE/6 -> Bus Creator18/6  "tuningStatus"
  inSOMANET_RKFE/1 -> Bus Creator18/1  "statusword"
  inSOMANET_LKFE/5 -> Bus Creator17/5  "userMISO"
  inSOMANET_RKFE/7 -> Bus Creator18/7  "errorSOMANET"
  inSOMANET_RKFE/8 -> Bus Creator18/8  "statusPhaseCurrentB"
  inSOMANET_RKFE/3 -> Bus Creator18/3  "actualVelocity"
  inSOMANET_RKFE/5 -> Bus Creator18/5  "userMISO"
  inSOMANET_LKFE/8 -> Bus Creator17/8  "statusPhaseCurrentB"
  inSOMANET_LKFE/12 -> Bus Creator17/12  "timestamp"
  Bus Creator17/1 -> [receivedFromLKFE]
  inSOMANET_RKFE/10 -> Bus Creator18/10  "opMode"
  inSOMANET_LKFE/6 -> Bus Creator17/6  "tuningStatus"
  inSOMANET_LKFE/10 -> Bus Creator17/10  "opMode"
  inSOMANET_RKFE/2 -> Bus Creator18/2  "actualAngle"
  inSOMANET_RKFE/9 -> Bus Creator18/9  "statusPhaseCurrentC"
  inSOMANET_RKFE/4 -> Bus Creator18/4  "actualTorque"
  inSOMANET_LKFE/9 -> Bus Creator17/9  "statusPhaseCurrentC"
  inSOMANET_LHFE/9 -> Bus Creator15/9  "statusPhaseCurrentC"
  inSOMANET_LKFE/7 -> Bus Creator17/7  "errorSOMANET"
  inSOMANET_LKFE/4 -> Bus Creator17/4  "actualTorque"
  MuxJointInfo/1 -> receivedFromSOMANETs/1
  inSOMANET_LKFE/3 -> Bus Creator17/3  "actualVelocity"
  inSOMANET_RHFE/8 -> Bus Creator16/8  "statusPhaseCurrentB"
  inSOMANET_RHFE/5 -> Bus Creator16/5  "userMISO"
  inSOMANET_LHFE/8 -> Bus Creator15/8  "statusPhaseCurrentB"
  inSOMANET_LHFE/4 -> Bus Creator15/4  "actualTorque"
  inSOMANET_LHFE/12 -> Bus Creator15/12  "timestamp"
  inSOMANET_LKFE/2 -> Bus Creator17/2  "actualAngle"
  inSOMANET_RHFE/12 -> Bus Creator16/12  "timestamp"
  inSOMANET_LHFE/3 -> Bus Creator15/3  "actualVelocity"
  inSOMANET_LKFE/1 -> Bus Creator17/1  "statusword"
  Bus Creator16/1 -> [receivedFromRHFE]
  Bus Creator15/1 -> [receivedFromLHFE]
  inSOMANET_RHFE/11 -> Bus Creator16/11  "statusTemperature"
  inSOMANET_LHFE/7 -> Bus Creator15/7  "errorSOMANET"
  inSOMANET_RHFE/10 -> Bus Creator16/10  "opMode"
  inSOMANET_RHFE/9 -> Bus Creator16/9  "statusPhaseCurrentC"
  inSOMANET_RHFE/7 -> Bus Creator16/7  "errorSOMANET"
  inSOMANET_RHFE/1 -> Bus Creator16/1  "statusword"
  inSOMANET_LHFE/2 -> Bus Creator15/2  "actualAngle"
  inSOMANET_RHFE/6 -> Bus Creator16/6  "tuningStatus"
  inSOMANET_RHFE/4 -> Bus Creator16/4  "actualTorque"
  inSOMANET_RHFE/3 -> Bus Creator16/3  "actualVelocity"
  inSOMANET_RHFE/2 -> Bus Creator16/2  "actualAngle"
  inSOMANET_LHFE/11 -> Bus Creator15/11  "statusTemperature"
  inSOMANET_LHFE/1 -> Bus Creator15/1  "statusword"
  inSOMANET_LHFE/10 -> Bus Creator15/10  "opMode"
  inSOMANET_LHFE/6 -> Bus Creator15/6  "tuningStatus"
  Bus Creator10/1 -> receivedFromPDB/1  "receivedFromPDB"
  inSOMANET_LHFE/5 -> Bus Creator15/5  "userMISO"
  "EtherCAT Init "/1 -> Terminator/1
  inSOMANET_LHFE/13 -> Bus Creator15/13  "actualMotorAngle"
  inSOMANET_LHFE/14 -> Bus Creator15/14  "actualMotorVelocity"
  inSOMANET_LKFE/13 -> Bus Creator17/13  "actualMotorAngle"
  inSOMANET_LKFE/14 -> Bus Creator17/14  "actualMotorVelocity"
  inSOMANET_RKFE/13 -> Bus Creator18/13  "actualMotorAngle"
  inSOMANET_RKFE/14 -> Bus Creator18/14  "actualMotorVelocity"
  inSOMANET_RHFE/13 -> Bus Creator16/13  "actualMotorAngle"
  inSOMANET_RHFE/14 -> Bus Creator16/14  "actualMotorVelocity"
  ReceiveFromBackGESv2s/1 -> receivedFromGESs/1
  ReceiveFromPDB/3 -> Bus Creator10/3  "errorMessagePDB"
  ReceiveFromPDB/4 -> Bus Creator10/4  "statusTemperatureDCDC"
  ReceiveFromPDB/5 -> Bus Creator10/5  "statusCurrentBattery"
  ReceiveFromPDB/6 -> Bus Creator10/6  "statusVoltageBattery"
  ReceiveFromPDB/2 -> Bus Creator10/2  "buttonPressedPDB"
  ReceiveFromInputDeviceDummy/1 -> receivedFromInputDevice/1  "desiredState"

== system HardwareCommunication/HardwareCommunicationFourJointsAndBuzzer/SendFourJoints ==
  sendToSOMANETs : Inport  OutDataTypeStr=Bus: EtherCATSendToSOMANET  PortDimensions=[1 4]  BusOutputAsStruct=on
  sendToInputDevice : Inport  Port=2  OutDataTypeStr=Bus: EtherCATSendToInputDevice  BusOutputAsStruct=on
  sendToGES : Inport  Port=3  BusOutputAsStruct=on
  sendToPDB : Inport  Port=4  OutDataTypeStr=Bus: EtherCATSendToPDB  BusOutputAsStruct=on
  DemuxJointInfo : VariousLibrary/DemuxJointInfo
  "SendToInputDeviceDummy " : SendToInputDevice/SendToInputDeviceDummy 
  SendToPDB : SendToPDB/SendToPDB
  SendToSomanetLHFE : SendToSOMANET/SendToSomanetLHFE
  SendToSomanetLKFE : SendToSOMANET/SendToSomanetLKFE
  SendToSomanetRHFE : SendToSOMANET/SendToSomanetRHFE
  SendToSomanetRKFE : SendToSOMANET/SendToSomanetRKFE
  sendToGES1 : SendToGES/sendToGES
  wires:
  sendToGES/1 -> sendToGES1/1
  DemuxJointInfo/4 -> SendToSomanetRKFE/1
  DemuxJointInfo/1 -> SendToSomanetLHFE/1
  DemuxJointInfo/2 -> SendToSomanetLKFE/1
  DemuxJointInfo/3 -> SendToSomanetRHFE/1
  sendToSOMANETs/1 -> DemuxJointInfo/1
  sendToPDB/1 -> SendToPDB/1
  sendToInputDevice/1 -> "SendToInputDeviceDummy "/1

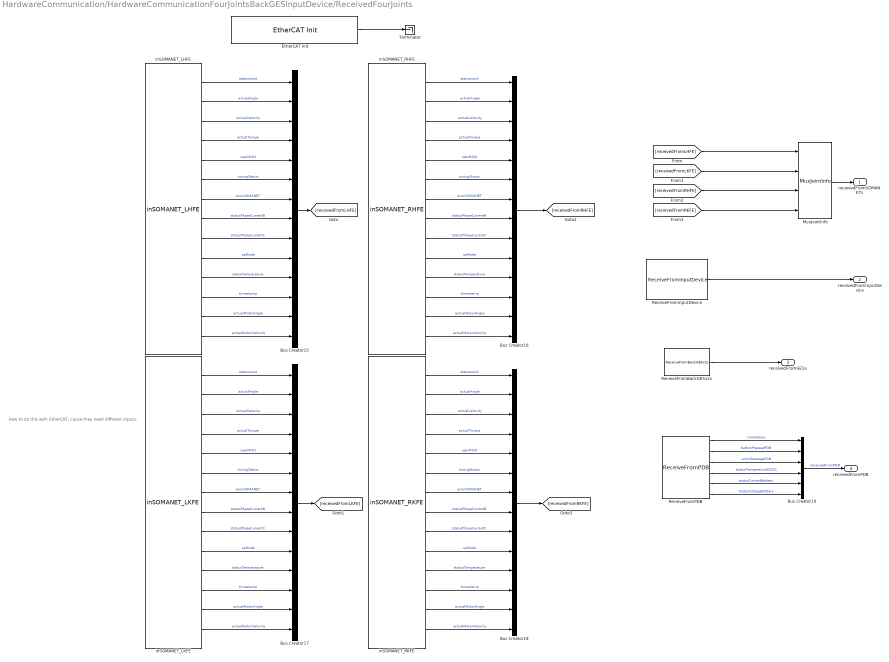
== system HardwareCommunication/HardwareCommunicationFourJointsBackGESInputDevice/ReceivedFourJoints ==
  note: How to do this with EtherCAT, cause they need different inputs.
  Bus Creator10 : BusCreator  Inputs=6  OutDataTypeStr=Bus: EtherCATReceivedFromPDB  NonVirtualBus=on
  Bus Creator{15..18} (4 alike) : BusCreator  Inputs=14  OutDataTypeStr=Bus: EtherCATReceivedFromSOMANET  NonVirtualBus=on
  "EtherCAT Init " : xpcethercatlib/EtherCAT Init   Priority=0  config_file=..\EcatXML\FourJointsBackGESInputDevice_eni.xml  device_id=0  pci_bus=2  pci_slot=0  dctuning=0  enaDebug=on  enaDC=on  errLink=on  masterDbg=on  stateChgDbg=on  baseClock=off  masterCfg=off  logFile='c:\dbglog.txt'  sample_time=0.002000  DCMode=0
  MuxJointInfo : VariousLibrary/MuxJointInfo
  ReceiveFromBackGESv2s : ReceiveFromGES/ReceiveFromBackGESv2s
  ReceiveFromInputDevice : ReceiveFromInputDevice/ReceiveFromInputDevice
  ReceiveFromPDB : ReceiveFromPDB/ReceiveFromPDB
  Terminator : Terminator
  inSOMANET_LHFE : inSOMANET/inSOMANET_LHFE
  inSOMANET_LKFE : inSOMANET/inSOMANET_LKFE
  inSOMANET_RHFE : inSOMANET/inSOMANET_RHFE
  inSOMANET_RKFE : inSOMANET/inSOMANET_RKFE
  receivedFromSOMANETs : Outport  OutDataTypeStr=Bus: EtherCATReceivedFromSOMANET  PortDimensions=[ 1 4 ]  BusOutputAsStruct=on
  receivedFromInputDevice : Outport  Port=2  OutDataTypeStr=Bus: EtherCATReceivedFromInputDevice  BusOutputAsStruct=on
  receivedFromGESs : Outport  Port=3  OutDataTypeStr=Bus: EtherCATReceivedFromGES  PortDimensions=[1 4]  BusOutputAsStruct=on
  receivedFromPDB : Outport  Port=4  OutDataTypeStr=Bus: EtherCATReceivedFromPDB  BusOutputAsStruct=on
  wires:
  ReceiveFromPDB/2 -> Bus Creator10/2  "buttonPressedPDB"
  ReceiveFromPDB/6 -> Bus Creator10/6  "statusVoltageBattery"
  ReceiveFromPDB/5 -> Bus Creator10/5  "statusCurrentBattery"
  ReceiveFromPDB/4 -> Bus Creator10/4  "statusTemperatureDCDC"
  ReceiveFromPDB/3 -> Bus Creator10/3  "errorMessagePDB"
  ReceiveFromBackGESv2s/1 -> receivedFromGESs/1
  inSOMANET_RHFE/14 -> Bus Creator16/14  "actualMotorVelocity"
  inSOMANET_RHFE/13 -> Bus Creator16/13  "actualMotorAngle"
  inSOMANET_RKFE/14 -> Bus Creator18/14  "actualMotorVelocity"
  inSOMANET_RKFE/13 -> Bus Creator18/13  "actualMotorAngle"
  inSOMANET_LKFE/14 -> Bus Creator17/14  "actualMotorVelocity"
  inSOMANET_LKFE/13 -> Bus Creator17/13  "actualMotorAngle"
  inSOMANET_LHFE/14 -> Bus Creator15/14  "actualMotorVelocity"
  inSOMANET_LHFE/13 -> Bus Creator15/13  "actualMotorAngle"
  "EtherCAT Init "/1 -> Terminator/1
  inSOMANET_LHFE/5 -> Bus Creator15/5  "userMISO"
  Bus Creator10/1 -> receivedFromPDB/1  "receivedFromPDB"
  inSOMANET_LHFE/6 -> Bus Creator15/6  "tuningStatus"
  inSOMANET_LHFE/10 -> Bus Creator15/10  "opMode"
  inSOMANET_LHFE/1 -> Bus Creator15/1  "statusword"
  inSOMANET_LHFE/11 -> Bus Creator15/11  "statusTemperature"
  inSOMANET_RHFE/2 -> Bus Creator16/2  "actualAngle"
  inSOMANET_RHFE/3 -> Bus Creator16/3  "actualVelocity"
  inSOMANET_RHFE/4 -> Bus Creator16/4  "actualTorque"
  inSOMANET_RHFE/6 -> Bus Creator16/6  "tuningStatus"
  inSOMANET_LHFE/2 -> Bus Creator15/2  "actualAngle"
  inSOMANET_RHFE/1 -> Bus Creator16/1  "statusword"
  inSOMANET_RHFE/7 -> Bus Creator16/7  "errorSOMANET"
  inSOMANET_RHFE/9 -> Bus Creator16/9  "statusPhaseCurrentC"
  inSOMANET_RHFE/10 -> Bus Creator16/10  "opMode"
  inSOMANET_LHFE/7 -> Bus Creator15/7  "errorSOMANET"
  inSOMANET_RHFE/11 -> Bus Creator16/11  "statusTemperature"
  Bus Creator15/1 -> [receivedFromLHFE]
  Bus Creator16/1 -> [receivedFromRHFE]
  inSOMANET_LKFE/1 -> Bus Creator17/1  "statusword"
  inSOMANET_LHFE/3 -> Bus Creator15/3  "actualVelocity"
  inSOMANET_RHFE/12 -> Bus Creator16/12  "timestamp"
  inSOMANET_LKFE/2 -> Bus Creator17/2  "actualAngle"
  inSOMANET_LHFE/12 -> Bus Creator15/12  "timestamp"
  inSOMANET_LHFE/4 -> Bus Creator15/4  "actualTorque"
  inSOMANET_LHFE/8 -> Bus Creator15/8  "statusPhaseCurrentB"
  inSOMANET_RHFE/5 -> Bus Creator16/5  "userMISO"
  inSOMANET_RHFE/8 -> Bus Creator16/8  "statusPhaseCurrentB"
  inSOMANET_LKFE/3 -> Bus Creator17/3  "actualVelocity"
  MuxJointInfo/1 -> receivedFromSOMANETs/1
  inSOMANET_LKFE/4 -> Bus Creator17/4  "actualTorque"
  inSOMANET_LKFE/7 -> Bus Creator17/7  "errorSOMANET"
  inSOMANET_LHFE/9 -> Bus Creator15/9  "statusPhaseCurrentC"
  inSOMANET_LKFE/9 -> Bus Creator17/9  "statusPhaseCurrentC"
  inSOMANET_RKFE/4 -> Bus Creator18/4  "actualTorque"
  inSOMANET_RKFE/9 -> Bus Creator18/9  "statusPhaseCurrentC"
  inSOMANET_RKFE/2 -> Bus Creator18/2  "actualAngle"
  inSOMANET_LKFE/10 -> Bus Creator17/10  "opMode"
  ReceiveFromInputDevice/1 -> receivedFromInputDevice/1
  inSOMANET_LKFE/6 -> Bus Creator17/6  "tuningStatus"
  inSOMANET_RKFE/10 -> Bus Creator18/10  "opMode"
  Bus Creator17/1 -> [receivedFromLKFE]
  inSOMANET_LKFE/12 -> Bus Creator17/12  "timestamp"
  inSOMANET_LKFE/8 -> Bus Creator17/8  "statusPhaseCurrentB"
  inSOMANET_RKFE/5 -> Bus Creator18/5  "userMISO"
  inSOMANET_RKFE/3 -> Bus Creator18/3  "actualVelocity"
  inSOMANET_RKFE/8 -> Bus Creator18/8  "statusPhaseCurrentB"
  inSOMANET_RKFE/7 -> Bus Creator18/7  "errorSOMANET"
  inSOMANET_LKFE/5 -> Bus Creator17/5  "userMISO"
  inSOMANET_RKFE/1 -> Bus Creator18/1  "statusword"
  inSOMANET_RKFE/6 -> Bus Creator18/6  "tuningStatus"
  inSOMANET_RKFE/12 -> Bus Creator18/12  "timestamp"
  inSOMANET_LKFE/11 -> Bus Creator17/11  "statusTemperature"
  inSOMANET_RKFE/11 -> Bus Creator18/11  "statusTemperature"
  Bus Creator18/1 -> [receivedFromRKFE]
  [receivedFromLHFE] -> MuxJointInfo/1
  [receivedFromRHFE] -> MuxJointInfo/3
  [receivedFromRKFE] -> MuxJointInfo/4
  [receivedFromLKFE] -> MuxJointInfo/2
  ReceiveFromPDB/1 -> Bus Creator10/1  "timestamp"

== system HardwareCommunication/HardwareCommunicationFourJointsBackGESInputDevice/SendFourJoints ==
  sendToSOMANETs : Inport  OutDataTypeStr=Bus: EtherCATSendToSOMANET  PortDimensions=[1 4]  BusOutputAsStruct=on
  sendToInputDevice : Inport  Port=2  OutDataTypeStr=Bus: EtherCATSendToInputDevice  BusOutputAsStruct=on
  sendToGES : Inport  Port=3  BusOutputAsStruct=on
  sendToPDB : Inport  Port=4  OutDataTypeStr=Bus: EtherCATSendToPDB  BusOutputAsStruct=on
  DemuxJointInfo : VariousLibrary/DemuxJointInfo
  SendToInputDevice : SendToInputDevice/SendToInputDevice
  SendToPDB : SendToPDB/SendToPDB
  SendToSomanetLHFE : SendToSOMANET/SendToSomanetLHFE
  SendToSomanetLKFE : SendToSOMANET/SendToSomanetLKFE
  SendToSomanetRHFE : SendToSOMANET/SendToSomanetRHFE
  SendToSomanetRKFE : SendToSOMANET/SendToSomanetRKFE
  sendToGES1 : SendToGES/sendToGES
  wires:
  sendToInputDevice/1 -> SendToInputDevice/1
  sendToPDB/1 -> SendToPDB/1
  sendToSOMANETs/1 -> DemuxJointInfo/1
  DemuxJointInfo/3 -> SendToSomanetRHFE/1
  DemuxJointInfo/2 -> SendToSomanetLKFE/1
  DemuxJointInfo/1 -> SendToSomanetLHFE/1
  DemuxJointInfo/4 -> SendToSomanetRKFE/1
  sendToGES/1 -> sendToGES1/1
